simulink model "ObjectTrackerHDL_ew"  (R2024b)
settings: Solver=VariableStepAuto  StartTime=0.0  StopTime=0.2  RelTol=1e-3  EnableMultiTasking=on
PreLoadFcn:
  | % Blank input
  | img = zeros(480,640);
  | 
  | % Initialize ROI and its center
  | ROI = [175 270 127 127];
  | center = [ROI(2)+(ROI(4)+1)/2 ROI(1)+(ROI(3)+1)/2];
  | 
  | % Template Size
  | templateSize = 128;
  | tSize = templateSize;
  | 
  | % Learning rate
  | eta = 0.075;
  | 
  | % Number of training images
  | trainCount = 2;
  | 
  | % Gaussian Variance
  | sig = 2;
  | 
  | % Generate a Gaussian centered on the first frame
  | iSize = size(img);
  | [x,y] = ndgrid(1:iSize(1), 1:iSize(2));
  | gauss = exp(-((x-center(1)).^2 + (y-center(2)).^2)./(2*sig));
  | gauss = mat2gray(gauss);
  | 
  | % Generate the first template
  | img = imcrop(img, ROI);
  | gauss = imcrop(gauss, ROI);
  | 
  | % Generate the preprocess windowing function
  | [w1,w2] = meshgrid(window(@hann,tSize),window(@hann,tSize));
  | win = w1.*w2;
  | 
  | % Blank initial coefficients
  | G = zeros(tSize,tSize);
  | Ai = zeros(tSize,tSize);
  | Bi = zeros(tSize,tSize);
  | Hi = zeros(tSize,tSize);
  | 
  | numRows = tSize;
  | numCols = tSize;
InitFcn:
  | % Read the first frame
  | vidFReader = VideoReader(get_param('ObjectTrackerHDL/Input','inputFilename'));
  | img = read(vidFReader,1);
  | if (size(img,3) == 3)
  |     img = rgb2gray(img);
  | end
  | img = double(img);
  | 
  | % Initialize Object Center
  | objectCenter = str2num(get_param('ObjectTrackerHDL/ObjectTrackerHDL','objectCenter'));
  | 
  | % Template Size
  | templateSize = str2num(get_param('ObjectTrackerHDL/ObjectTrackerHDL','templateSize'));
  | originROI = objectCenter-templateSize/2;
  | tSize = templateSize;
  | 
  | % Initialize ROI and its center
  | ROI = [originROI tSize-1 tSize-1];
  | center = [ROI(2)+(ROI(4)+1)/2 ROI(1)+(ROI(3)+1)/2];
  | 
  | % Learning rate
  | eta = 0.075;
  | 
  | % Number of training images
  | trainCount = 128;
  | 
  | % Gaussian Variance
  | sig = 2;
  | 
  | % Generate a Gaussian centered on the first frame
  | iSize = size(img);
  | [x,y] = ndgrid(1:iSize(1), 1:iSize(2));
  | gauss = exp(-((x-center(1)).^2 + (y-center(2)).^2)./(2*sig));
  | gauss = mat2gray(gauss);
  | 
  | % Generate the first template
  | img = imcrop(img, ROI);
  | gauss = imcrop(gauss, ROI);
  | 
  | % Generate the preprocess windowing function
  | [w1,w2] = meshgrid(window(@hann,tSize),window(@hann,tSize));
  | win = w1.*w2;
  | 
  | % Preprocessing the first template
  | hgamma = vision.GammaCorrector(2.0,'Correction','De-gamma');
  | img = hgamma(uint8(img));
  | img = double(img);
  | mean1 = mean(img(:));
  | std1 = std(img(:));
  | img = (img-mean1)/std1;
  | fii = img.*win;
  | 
  | % Convert to frequency domain and calculate initial coefficients
  | G = fft2(gauss);
  | Ai = (G.*conj(fft2(fii)));
  | Bi = real((fft2(fii).*conj(fft2(fii))));
  | 
  | rng('default');
  | % Initial training procedure
  | for i = 1:trainCount
  | ... (+19 lines)
model workspace (MAT data in the model file):
  mwTaskManagerKernelLatency = 0
undefined symbols (not defined in the file): a, b, c, Rec, SDTV
libraries: hdlsllib x61, simulink x17, visionhdlutilities x8, visionstatistics x6, dsphdlxfrm2 x6, visionconversions x4, visiontransforms x3, visionhdlio x2, visionhdlconversions x2, visionhdlstatistics x2, visionanalysis x2, visionsinks x1
(part 2 of 3)

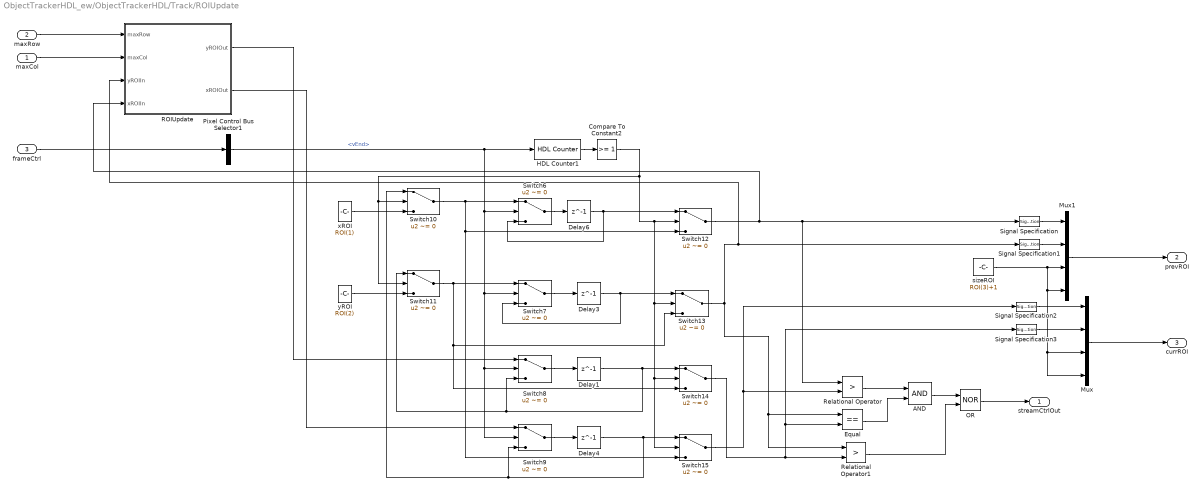
== system ObjectTrackerHDL_ew/ObjectTrackerHDL/Track/ROIUpdate ==
  maxCol : Inport
  maxRow : Inport  Port=2
  frameCtrl : Inport  Port=3
  AND : Logic  AllPortsSameDT=off  OutDataTypeStr=boolean
  Compare To Constant2 : simulink/Logic and Bit Operations/Compare To Constant  relop=>=  const=1  OutDataTypeStr=boolean
  Delay{1,3..4,6} (4 alike) : Delay  DelayLength=1
  Equal : RelationalOperator  Operator===  OutDataTypeStr=boolean  RndMeth=Simplest  InputSameDT=off
  HDL Counter1 : hdlsllib/Sources/HDL Counter  CountType=Count limited  CountInit=0  CountStep=1  CountMax=4095  CountFromType=Initial value  CountFrom=0  CountResetPort=off  CountLoadPort=off  CountEnbPort=on  CountDirPort=off  CountHitOutputPort=off  CountDataType=Unsigned  CountWordLen=12  CountFracLen=0  CountSampTime=1
  Mux : Mux
  Mux1 : Mux
  OR : Logic  Operator=NOR  AllPortsSameDT=off  OutDataTypeStr=boolean
  Pixel Control Bus Selector1 : BusSelector  OutputSignals=vEnd
  ROIUpdate : Subsystem
  Relational Operator : RelationalOperator  Operator=>  OutDataTypeStr=boolean  RndMeth=Simplest  InputSameDT=off
  Relational Operator1 : RelationalOperator  Operator=>  OutDataTypeStr=boolean  RndMeth=Simplest  InputSameDT=off
  Signal Specification{,1..3} (4 alike) : SignalSpecification  Dimensions=1
  Switch{6..15} (10 alike) : Switch  Criteria=u2 ~= 0  SaturateOnIntegerOverflow=off  InputSameDT=off
  sizeROI : Constant  Value=ROI(3)+1  OutDataTypeStr=uint16  SampleTime=-1
  xROI : Constant  Value=ROI(1)  OutDataTypeStr=uint16  SampleTime=-1
  yROI : Constant  Value=ROI(2)  OutDataTypeStr=uint16  SampleTime=-1
  streamCtrlOut : Outport
  prevROI : Outport  Port=2
  currROI : Outport  Port=3
  wires:
  Signal Specification/1 -> Mux1/1
  Switch15/1 -> Signal Specification2/1, Relational Operator/2
  Pixel Control Bus Selector1/1 -> Switch9/2, Switch8/2, Switch7/2, Switch6/2, HDL Counter1/1  "<vEnd>"
  Switch13/1 -> ROIUpdate/3(yROIIn), Signal Specification1/1, Equal/1, Relational Operator1/1
  Relational Operator/1 -> AND/1
  Signal Specification1/1 -> Mux1/2
  Switch12/1 -> ROIUpdate/4(xROIIn), Signal Specification/1, Relational Operator/1
  xROI/1 -> Switch10/3
  AND/1 -> OR/1
  Signal Specification3/1 -> Mux/2
  yROI/1 -> Switch11/3
  Switch14/1 -> Signal Specification3/1, Equal/2, Relational Operator1/2
  HDL Counter1/1 -> Compare To Constant2/1
  Equal/1 -> AND/2
  Signal Specification2/1 -> Mux/1
  Switch10/1 -> Switch15/3, Switch12/3, Switch6/1
  Relational Operator1/1 -> OR/2
  OR/1 -> streamCtrlOut/1
  maxRow/1 -> ROIUpdate/1(maxRow)
  maxCol/1 -> ROIUpdate/2(maxCol)
  Mux1/1 -> prevROI/1
  Mux/1 -> currROI/1
  Switch11/1 -> Switch14/3, Switch13/3, Switch7/1
  sizeROI/1 -> Mux/3, Mux/4, Mux1/4, Mux1/3
  Switch6/1 -> Delay6/1
  Switch7/1 -> Delay3/1
  Switch8/1 -> Delay1/1
  Switch9/1 -> Delay4/1
  Compare To Constant2/1 -> Switch12/2, Switch13/2, Switch15/2, Switch14/2, Switch11/2, Switch10/2
  frameCtrl/1 -> Pixel Control Bus Selector1/1
  Delay6/1 -> Switch6/3, Switch12/1
  Delay3/1 -> Switch7/3, Switch13/1
  Delay1/1 -> Switch8/3, Switch11/1, Switch14/1
  Delay4/1 -> Switch10/1, Switch9/3, Switch15/1
  ROIUpdate/2(xROIOut) -> Switch9/1
  ROIUpdate/1(yROIOut) -> Switch8/1

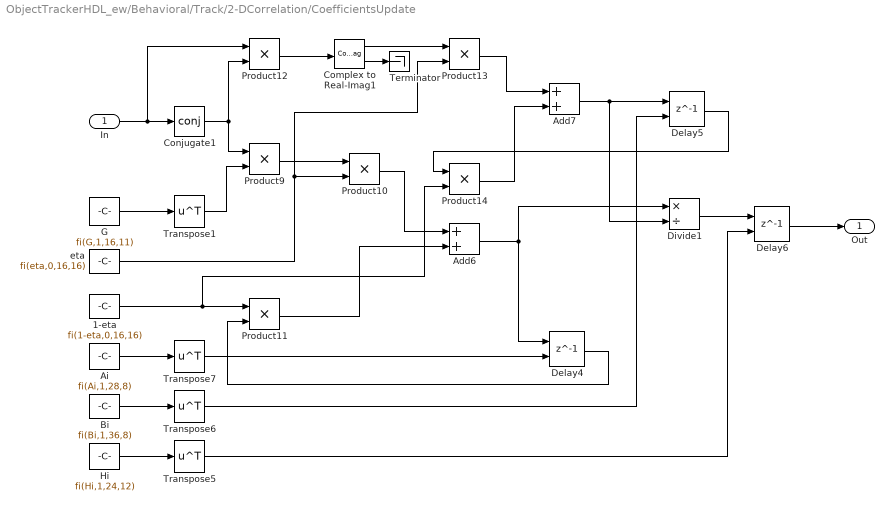
== system ObjectTrackerHDL_ew/Behavioral/Track/2-DCorrelation/CoefficientsUpdate ==
  In : Inport
  1-eta : Constant  Value=fi(1-eta,0,16,16)  OutDataTypeStr=fixdt(0,16,16)  SampleTime=-1
  Add6 : Sum  OutDataTypeStr=fixdt(1,28,8)
  Add7 : Sum  OutDataTypeStr=fixdt(1,36,8)
  Ai : Constant  Value=fi(Ai,1,28,8)  OutDataTypeStr=fixdt(1,28,8)  SampleTime=-1
  Bi : Constant  Value=fi(Bi,1,36,8)  OutDataTypeStr=fixdt(1,36,8)  SampleTime=-1
  Complex to Real-Imag1 : ComplexToRealImag
  Conjugate1 : Math  Operator=conj  SignedPower=on  RndMeth=Zero
  Delay4 : Delay  DelayLength=1  InitialConditionSource=Input port  InitialCondition=Ai
      settings: InputPortMap=u0,p4
  Delay5 : Delay  DelayLength=1  InitialConditionSource=Input port  InitialCondition=Bi
      settings: InputPortMap=u0,p4
  Delay6 : Delay  DelayLength=1  InitialConditionSource=Input port  InitialCondition=Hi
      settings: InputPortMap=u0,p4
  Divide1 : Product  Inputs=*/  OutDataTypeStr=fixdt(1,24,12)  RndMeth=Simplest  SaturateOnIntegerOverflow=on
  G : Constant  Value=fi(G,1,16,11)  VectorParams1D=off  SampleTime=-1
  Hi : Constant  Value=fi(Hi,1,24,12)  OutDataTypeStr=fixdt(1,24,12)  SampleTime=-1
  Product10 : Product  OutDataTypeStr=fixdt(1,24,12)
  Product11 : Product  OutDataTypeStr=fixdt(1,28,8)
  Product12 : Product  OutDataTypeStr=fixdt(1,32,8)
  Product13 : Product  OutDataTypeStr=fixdt(1,32,12)
  Product14 : Product  OutDataTypeStr=fixdt(1,36,8)
  Product9 : Product  OutDataTypeStr=fixdt(1,24,8)
  Terminator : Terminator
  Transpose{1,5..7} (4 alike) : Math  Operator=transpose
  eta : Constant  Value=fi(eta,0,16,16)  SampleTime=-1
  Out : Outport
  wires:
  Product14/1 -> Add7/2
  Ai/1 -> Transpose7/1
  Add6/1 -> Delay4/1, Divide1/1
  Divide1/1 -> Delay6/1
  eta/1 -> Product13/2, Product10/2
  In/1 -> Product12/1, Conjugate1/1
  Product9/1 -> Product10/1
  Conjugate1/1 -> Product12/2, Product9/1
  Product11/1 -> Add6/2
  1-eta/1 -> Product11/1, Product14/2
  Transpose6/1 -> Delay5/2
  Add7/1 -> Delay5/1, Divide1/2
  Hi/1 -> Transpose5/1
  Product10/1 -> Add6/1
  Delay5/1 -> Product14/1
  Product13/1 -> Add7/1
  G/1 -> Transpose1/1
  Complex to Real-Imag1/2 -> Terminator/1
  Complex to Real-Imag1/1 -> Product13/1
  Delay6/1 -> Out/1
  Bi/1 -> Transpose6/1
  Product12/1 -> Complex to Real-Imag1/1
  Transpose5/1 -> Delay6/2
  Transpose7/1 -> Delay4/2
  Delay4/1 -> Product11/2
  Transpose1/1 -> Product9/2

== system ObjectTrackerHDL_ew/Behavioral/Track/ROIUpdate/CurrValidROI ==
  ROIIn : Inport
  Constant : Constant  Value=iSize(1)-tSize  OutDataTypeStr=uint16  SampleTime=-1
  Constant1 : Constant  Value=iSize(2)-tSize  OutDataTypeStr=uint16  SampleTime=-1
  Demux : Demux
  Mux1 : Mux
  Relational Operator : RelationalOperator  Operator=<  OutDataTypeStr=boolean  RndMeth=Simplest  InputSameDT=off
  Relational Operator1 : RelationalOperator  Operator=<  OutDataTypeStr=boolean  RndMeth=Simplest  InputSameDT=off
  Switch : Switch  Criteria=u2 ~= 0  SaturateOnIntegerOverflow=off  InputSameDT=off
  Switch1 : Switch  Criteria=u2 ~= 0  SaturateOnIntegerOverflow=off  InputSameDT=off
  ROIOut : Outport
  wires:
  Mux1/1 -> ROIOut/1
  ROIIn/1 -> Demux/1
  Demux/1 -> Switch/1, Relational Operator/1
  Constant1/1 -> Switch/3, Relational Operator/2
  Demux/2 -> Relational Operator1/1, Switch1/1
  Constant/1 -> Switch1/3, Relational Operator1/2
  Demux/3 -> Mux1/3
  Demux/4 -> Mux1/4
  Relational Operator/1 -> Switch/2
  Switch/1 -> Mux1/1
  Relational Operator1/1 -> Switch1/2
  Switch1/1 -> Mux1/2

== system ObjectTrackerHDL_ew/Behavioral/Track/ROIUpdate/PrevValidROI ==
  ROIIn : Inport
  Constant : Constant  Value=iSize(1)-tSize  OutDataTypeStr=uint16  SampleTime=-1
  Constant1 : Constant  Value=iSize(2)-tSize  OutDataTypeStr=uint16  SampleTime=-1
  Demux : Demux
  Mux1 : Mux
  Relational Operator : RelationalOperator  Operator=<  OutDataTypeStr=boolean  RndMeth=Simplest  InputSameDT=off
  Relational Operator1 : RelationalOperator  Operator=<  OutDataTypeStr=boolean  RndMeth=Simplest  InputSameDT=off
  Switch : Switch  Criteria=u2 ~= 0  SaturateOnIntegerOverflow=off  InputSameDT=off
  Switch1 : Switch  Criteria=u2 ~= 0  SaturateOnIntegerOverflow=off  InputSameDT=off
  ROIOut : Outport
  wires:
  Mux1/1 -> ROIOut/1
  ROIIn/1 -> Demux/1
  Demux/1 -> Switch/1, Relational Operator/1
  Constant1/1 -> Switch/3, Relational Operator/2
  Demux/2 -> Relational Operator1/1, Switch1/1
  Constant/1 -> Switch1/3, Relational Operator1/2
  Demux/3 -> Mux1/3
  Demux/4 -> Mux1/4
  Relational Operator/1 -> Switch/2
  Switch/1 -> Mux1/1
  Relational Operator1/1 -> Switch1/2
  Switch1/1 -> Mux1/2

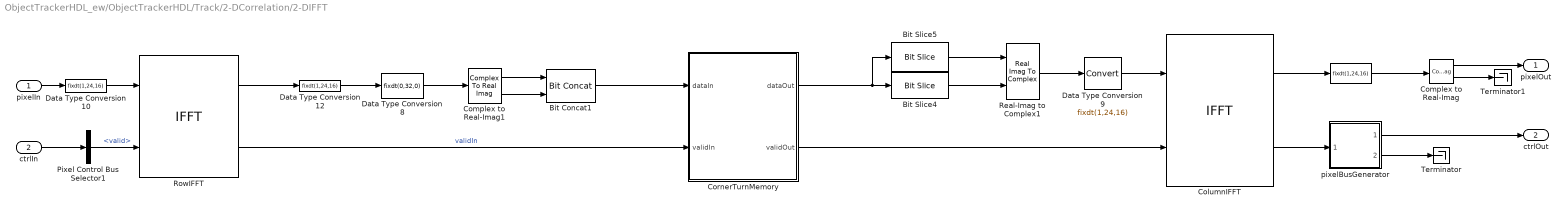
== system ObjectTrackerHDL_ew/ObjectTrackerHDL/Track/2-DCorrelation/2-DIFFT ==
  pixelIn : Inport
  ctrlIn : Inport  Port=2
  " " : DataTypeConversion  OutDataTypeStr=fixdt(1,24,16)  SaturateOnIntegerOverflow=off  RndMeth=Floor
  Bit Concat1 : hdlsllib/Logic and Bit Operations/Bit Concat  numInputs=2
  Bit Slice4 : hdlsllib/Logic and Bit Operations/Bit Slice  lidx=31  ridx=0
  Bit Slice5 : hdlsllib/Logic and Bit Operations/Bit Slice  lidx=63  ridx=32
  ColumnIFFT : dsphdlxfrm2/IFFT  Architecture=Streaming Radix 2^2  FFTLengthSource=Property  FFTLength=tSize  FFTLengthMax=1024  ComplexMultiplication=Use 4 multipliers and 2 adders  BitReversedOutput=off  BitReversedInput=off  Normalize=on  SimulateUsing=Code generation  RoundingMethod=Floor  ResetInputPort=off  StartOutputPort=off  EndOutputPort=off
  Complex to Real-Imag : ComplexToRealImag
  Complex to Real-Imag1 : ComplexToRealImag
  CornerTurnMemory : Subsystem
  Data Type Conversion10 : DataTypeConversion  OutDataTypeStr=fixdt(1,24,16)  SaturateOnIntegerOverflow=off  RndMeth=Floor
  Data Type Conversion12 : DataTypeConversion  OutDataTypeStr=fixdt(1,24,16)  SaturateOnIntegerOverflow=off  RndMeth=Floor
  Data Type Conversion8 : DataTypeConversion  OutDataTypeStr=fixdt(0,32,0)  ConvertRealWorld=Stored Integer (SI)  SaturateOnIntegerOverflow=off  RndMeth=Floor
  Data Type Conversion9 : DataTypeConversion  OutDataTypeStr=fixdt(1,24,16)  ConvertRealWorld=Stored Integer (SI)  SaturateOnIntegerOverflow=off  RndMeth=Floor
  Pixel Control Bus Selector1 : BusSelector  OutputSignals=valid
  Real-Imag to Complex1 : RealImagToComplex
  RowIFFT : dsphdlxfrm2/IFFT  Architecture=Streaming Radix 2^2  FFTLengthSource=Property  FFTLength=tSize  FFTLengthMax=1024  ComplexMultiplication=Use 4 multipliers and 2 adders  BitReversedOutput=off  BitReversedInput=off  Normalize=on  SimulateUsing=Code generation  RoundingMethod=Floor  ResetInputPort=off  StartOutputPort=off  EndOutputPort=off
  Terminator : Terminator
  Terminator1 : Terminator
  pixelBusGenerator : Subsystem  mask{hEnd=tSize - 1, vEnd=tSize * tSize - 1}
      mask prompts: hEnd "hEnd Count"; vEnd "vEnd Count"
      mask DialogControl DescGroupVar Prompt: Counter Values
  pixelOut : Outport
  ctrlOut : Outport  Port=2
  wires:
  Bit Slice4/1 -> Real-Imag to Complex1/2
  Complex to Real-Imag1/1 -> Bit Concat1/1
  pixelIn/1 -> Data Type Conversion10/1
  Data Type Conversion12/1 -> Data Type Conversion8/1
  Data Type Conversion8/1 -> Complex to Real-Imag1/1
  Data Type Conversion10/1 -> RowIFFT/1
  ColumnIFFT/1 -> " "/1
  ctrlIn/1 -> Pixel Control Bus Selector1/1
  pixelBusGenerator/2(frameDone) -> Terminator/1
  RowIFFT/1 -> Data Type Conversion12/1
  Complex to Real-Imag1/2 -> Bit Concat1/2
  ColumnIFFT/2 -> pixelBusGenerator/1(validIn)
  Data Type Conversion9/1 -> ColumnIFFT/1
  Bit Slice5/1 -> Real-Imag to Complex1/1
  Real-Imag to Complex1/1 -> Data Type Conversion9/1
  pixelBusGenerator/1(busOut) -> ctrlOut/1
  " "/1 -> Complex to Real-Imag/1
  Complex to Real-Imag/1 -> pixelOut/1
  Complex to Real-Imag/2 -> Terminator1/1
  Pixel Control Bus Selector1/1 -> RowIFFT/2  "<valid>"
  CornerTurnMemory/1(dataOut) -> Bit Slice5/1, Bit Slice4/1
  Bit Concat1/1 -> CornerTurnMemory/1(dataIn)
  RowIFFT/2 -> CornerTurnMemory/2(validIn)  "validIn"
  CornerTurnMemory/2(validOut) -> ColumnIFFT/2

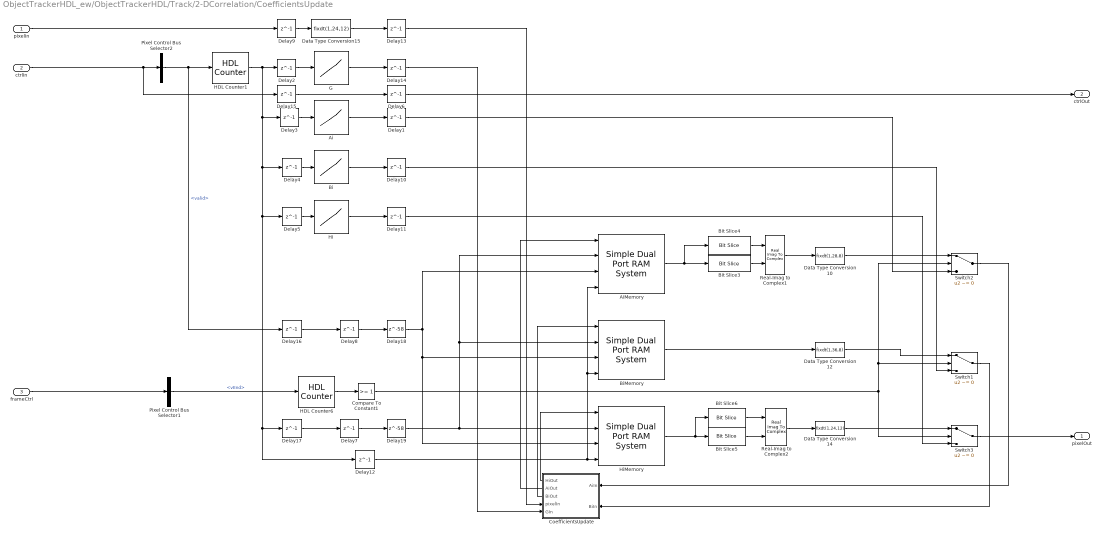
== system ObjectTrackerHDL_ew/ObjectTrackerHDL/Track/2-DCorrelation/CoefficientsUpdate ==
  pixelIn : Inport
  ctrlIn : Inport  Port=2
  frameCtrl : Inport  Port=3
  Ai : Lookup_n-D  NumberOfTableDimensions=1  LookupTableObject=''  BreakpointsForDimension1=[0:tSize * tSize - 1]  BreakpointsForDimension1FirstPoint=10  BreakpointsForDimension2FirstPoint=10  BreakpointsForDimension1Spacing=12  BreakpointsForDimension2Spacing=12  IndexSearchMethod=Evenly spaced points  Table=fi(Ai(:),1,28,8)  InterpMethod=Flat  DiagnosticForOutOfRangeInput=Error  InternalRulePriority=Speed  OutDataTypeStr=fixdt(1,28,8)  RndMeth=Simplest
  AiMemory : hdlsllib/HDL RAMs/Simple Dual Port RAM System  RAMType=Simple dual port  AsyncRead=off  WriteOutputValue=New data  RAMInitialValue=0  allowBusInputs=off  WritesHaveOutput=on  NumReads=0  NumWrites=1  SimulateUsing=Code generation  ModelRAMDelay=on
  Bi : Lookup_n-D  NumberOfTableDimensions=1  LookupTableObject=''  BreakpointsForDimension1=[0:tSize * tSize - 1]  BreakpointsForDimension1FirstPoint=10  BreakpointsForDimension2FirstPoint=10  BreakpointsForDimension1Spacing=12  BreakpointsForDimension2Spacing=12  IndexSearchMethod=Evenly spaced points  Table=fi(Bi(:),1,36,8)  InterpMethod=Flat  DiagnosticForOutOfRangeInput=Error  InternalRulePriority=Speed  OutDataTypeStr=fixdt(1,36,8)  RndMeth=Simplest
  BiMemory : hdlsllib/HDL RAMs/Simple Dual Port RAM System  RAMType=Simple dual port  AsyncRead=off  WriteOutputValue=New data  RAMInitialValue=0  allowBusInputs=off  WritesHaveOutput=on  NumReads=0  NumWrites=1  SimulateUsing=Code generation  ModelRAMDelay=on
  Bit Slice3 : hdlsllib/Logic and Bit Operations/Bit Slice  lidx=31  ridx=0
  Bit Slice4 : hdlsllib/Logic and Bit Operations/Bit Slice  lidx=63  ridx=32
  Bit Slice5 : hdlsllib/Logic and Bit Operations/Bit Slice  lidx=31  ridx=0
  Bit Slice6 : hdlsllib/Logic and Bit Operations/Bit Slice  lidx=63  ridx=32
  CoefficientsUpdate : Subsystem
      settings: PortSchema="{\"entries\":[{\"content\":{\"sides\":[{\"content\":{\"connectorIds\":[\"Out1\",\"Out2\",\"Out3\",\"In1\",\"In2\"]},\"type\":\"ConnectorPlacement.EquallySpacedRectSide\",\"uuid\":\"191c5b09-aed9-4d47-87b5-72a6c40c9cca\"},{\"content\":{\"connectorIds\":[\"In3\",\"In4\"],\"side\":\"RIGHT\"},\"type\":\"ConnectorPlacement.EquallySpacedRectSide\",\"uuid\":\"decd93cb-43a4-41cc-87f2-68ffa8f89900\"},{\"content\":{\"side\":\"TOP\"},\"type\":\"ConnectorPlacement.EquallySpacedRectSide\",\"uuid\":\"0d8c8ea6-6c17-441a-9a0f-239b887dcd47\"}]},\"type\":\"ConnectorPlacement.EquallySpacedConnector\",\"uuid\":\"0ec76fdc-f9ed-4753-8274-de70c3f7ff2d\"}],\"packageUris\":[\"http://schema.mathworks.com/mf0/Connector/R2020b\"],\"version\":\"1.0\"}"
  Compare To Constant1 : simulink/Logic and Bit Operations/Compare To Constant  relop=>=  const=1  OutDataTypeStr=boolean
  Data Type Conversion10 : DataTypeConversion  OutDataTypeStr=fixdt(1,28,8)  ConvertRealWorld=Stored Integer (SI)  SaturateOnIntegerOverflow=off  RndMeth=Floor
  Data Type Conversion12 : DataTypeConversion  OutDataTypeStr=fixdt(1,36,8)  ConvertRealWorld=Stored Integer (SI)  SaturateOnIntegerOverflow=off  RndMeth=Floor
  Data Type Conversion14 : DataTypeConversion  OutDataTypeStr=fixdt(1,24,12)  ConvertRealWorld=Stored Integer (SI)  SaturateOnIntegerOverflow=off  RndMeth=Floor
  Data Type Conversion15 : DataTypeConversion  OutDataTypeStr=fixdt(1,24,12)  SaturateOnIntegerOverflow=off  RndMeth=Floor
  Delay{1..17} (17 alike) : Delay  DelayLength=1
  Delay18 : Delay  DelayLength=58
  Delay19 : Delay  DelayLength=58
  G : Lookup_n-D  NumberOfTableDimensions=1  LookupTableObject=''  BreakpointsForDimension1=[0:tSize * tSize - 1]  BreakpointsForDimension1FirstPoint=10  BreakpointsForDimension2FirstPoint=10  BreakpointsForDimension1Spacing=12  BreakpointsForDimension2Spacing=12  IndexSearchMethod=Evenly spaced points  Table=fi(G(:),1,16,11)  InterpMethod=Flat  DiagnosticForOutOfRangeInput=Error  InternalRulePriority=Speed  OutDataTypeStr=fixdt(1,16,11)  RndMeth=Simplest
  HDL Counter1 : hdlsllib/Sources/HDL Counter  CountType=Count limited  CountInit=0  CountStep=1  CountMax=tSize * tSize - 1  CountFromType=Initial value  CountFrom=0  CountResetPort=off  CountLoadPort=off  CountEnbPort=on  CountDirPort=off  CountHitOutputPort=off  CountDataType=Unsigned  CountWordLen=ceil(log2(tSize * tSize - 1))  CountFracLen=0  CountSampTime=1
  HDL Counter6 : hdlsllib/Sources/HDL Counter  CountType=Count limited  CountInit=0  CountStep=1  CountMax=4095  CountFromType=Initial value  CountFrom=0  CountResetPort=off  CountLoadPort=off  CountEnbPort=on  CountDirPort=off  CountHitOutputPort=off  CountDataType=Unsigned  CountWordLen=12  CountFracLen=0  CountSampTime=1
  Hi : Lookup_n-D  NumberOfTableDimensions=1  LookupTableObject=''  BreakpointsForDimension1=[0:tSize * tSize - 1]  BreakpointsForDimension1FirstPoint=10  BreakpointsForDimension2FirstPoint=10  BreakpointsForDimension1Spacing=12  BreakpointsForDimension2Spacing=12  IndexSearchMethod=Evenly spaced points  Table=fi(Hi(:),1,24,12)  InterpMethod=Flat  DiagnosticForOutOfRangeInput=Error  InternalRulePriority=Speed  OutDataTypeStr=fixdt(1,24,12)  RndMeth=Simplest
  HiMemory : hdlsllib/HDL RAMs/Simple Dual Port RAM System  RAMType=Simple dual port  AsyncRead=off  WriteOutputValue=New data  RAMInitialValue=0  allowBusInputs=off  WritesHaveOutput=on  NumReads=0  NumWrites=1  SimulateUsing=Code generation  ModelRAMDelay=on
  Pixel Control Bus Selector1 : BusSelector  OutputSignals=vEnd
  Pixel Control Bus Selector2 : BusSelector  OutputSignals=valid
  Real-Imag to Complex1 : RealImagToComplex
  Real-Imag to Complex2 : RealImagToComplex
  Switch1 : Switch  Criteria=u2 ~= 0  SaturateOnIntegerOverflow=off  InputSameDT=off
  Switch2 : Switch  Criteria=u2 ~= 0  SaturateOnIntegerOverflow=off  InputSameDT=off
  Switch3 : Switch  Criteria=u2 ~= 0  SaturateOnIntegerOverflow=off  InputSameDT=off
  pixelOut : Outport
  ctrlOut : Outport  Port=2
  wires:
  Delay7/1 -> Delay19/1
  Data Type Conversion12/1 -> Switch1/1
  Bit Slice5/1 -> Real-Imag to Complex2/2
  AiMemory/1 -> Bit Slice4/1, Bit Slice3/1
  Pixel Control Bus Selector2/1 -> HDL Counter1/1, Delay16/1  "<valid>"
  Real-Imag to Complex1/1 -> Data Type Conversion10/1
  Bit Slice4/1 -> Real-Imag to Complex1/1
  Bit Slice3/1 -> Real-Imag to Complex1/2
  BiMemory/1 -> Data Type Conversion12/1
  Data Type Conversion10/1 -> Switch2/1
  HDL Counter6/1 -> Compare To Constant1/1
  Bit Slice6/1 -> Real-Imag to Complex2/1
  Real-Imag to Complex2/1 -> Data Type Conversion14/1
  Data Type Conversion15/1 -> Delay13/1
  G/1 -> Delay14/1
  Switch2/1 -> CoefficientsUpdate/3(AiIn)
  Switch1/1 -> CoefficientsUpdate/4(BiIn)
  Pixel Control Bus Selector1/1 -> HDL Counter6/1  "<vEnd>"
  HiMemory/1 -> Bit Slice5/1, Bit Slice6/1
  Compare To Constant1/1 -> Switch3/2, Switch2/2, Switch1/2
  Data Type Conversion14/1 -> Switch3/1
  Delay8/1 -> Delay18/1
  Delay2/1 -> G/1
  Delay3/1 -> Ai/1
  Delay4/1 -> Bi/1
  Delay5/1 -> Hi/1
  Delay6/1 -> ctrlOut/1
  Delay9/1 -> Data Type Conversion15/1
  ctrlIn/1 -> Delay15/1, Pixel Control Bus Selector2/1
  pixelIn/1 -> Delay9/1
  frameCtrl/1 -> Pixel Control Bus Selector1/1
  CoefficientsUpdate/1(HiOut) -> HiMemory/1
  CoefficientsUpdate/3(BiOut) -> BiMemory/1
  CoefficientsUpdate/2(AiOut) -> AiMemory/1
  HDL Counter1/1 -> Delay12/1, Delay17/1, Delay5/1, Delay4/1, Delay3/1, Delay2/1
  Switch3/1 -> pixelOut/1
  Hi/1 -> Delay11/1
  Bi/1 -> Delay10/1
  Ai/1 -> Delay1/1
  Delay1/1 -> Switch2/3
  Delay10/1 -> Switch1/3
  Delay11/1 -> Switch3/3
  Delay12/1 -> HiMemory/4, AiMemory/4, BiMemory/4
  Delay13/1 -> CoefficientsUpdate/1(pixelIn)
  Delay14/1 -> CoefficientsUpdate/2(GIn)
  Delay15/1 -> Delay6/1
  Delay16/1 -> Delay8/1
  Delay17/1 -> Delay7/1
  Delay18/1 -> BiMemory/3, HiMemory/3, AiMemory/3
  Delay19/1 -> AiMemory/2, BiMemory/2, HiMemory/2

== system ObjectTrackerHDL_ew/ObjectTrackerHDL/Track/2-DCorrelation/Curr2-DFFT ==
  pixelIn : Inport
  ctrlIn : Inport  Port=2
  " " : DataTypeConversion  OutDataTypeStr=fixdt(1,24,12)  SaturateOnIntegerOverflow=off  RndMeth=Floor
  Bit Concat : hdlsllib/Logic and Bit Operations/Bit Concat  numInputs=2
  Bit Slice1 : hdlsllib/Logic and Bit Operations/Bit Slice  lidx=31  ridx=0
  Bit Slice2 : hdlsllib/Logic and Bit Operations/Bit Slice  lidx=63  ridx=32
  ColumnFFT : dsphdlxfrm2/FFT  Architecture=Streaming Radix 2^2  FFTLengthSource=Property  FFTLength=tSize  FFTLengthMax=1024  ComplexMultiplication=Use 4 multipliers and 2 adders  BitReversedOutput=off  BitReversedInput=off  Normalize=off  SimulateUsing=Code generation  RoundingMethod=Floor  ResetInputPort=off  StartOutputPort=off  EndOutputPort=off
  Complex to Real-Imag1 : ComplexToRealImag
  CornerTurnMemory : Subsystem
  Data Type Conversion2 : DataTypeConversion  OutDataTypeStr=fixdt(0,32,0)  ConvertRealWorld=Stored Integer (SI)  SaturateOnIntegerOverflow=off  RndMeth=Floor
  Data Type Conversion3 : DataTypeConversion  OutDataTypeStr=fixdt(1,28,16)  ConvertRealWorld=Stored Integer (SI)  SaturateOnIntegerOverflow=off  RndMeth=Floor
  Data Type Conversion6 : DataTypeConversion  OutDataTypeStr=fixdt(1,28,16)  SaturateOnIntegerOverflow=off  RndMeth=Floor
  Pixel Control Bus Selector1 : BusSelector  OutputSignals=valid
  Real-Imag to Complex : RealImagToComplex
  RowFFT : dsphdlxfrm2/FFT  Architecture=Streaming Radix 2^2  FFTLengthSource=Property  FFTLength=tSize  FFTLengthMax=1024  ComplexMultiplication=Use 4 multipliers and 2 adders  BitReversedOutput=off  BitReversedInput=off  Normalize=off  SimulateUsing=Code generation  RoundingMethod=Floor  ResetInputPort=off  StartOutputPort=off  EndOutputPort=off
  Terminator : Terminator
  pixelBusGenerator : Subsystem  mask{hEnd=tSize - 1, vEnd=tSize * tSize - 1}
      mask prompts: hEnd "hEnd Count"; vEnd "vEnd Count"
      mask DialogControl DescGroupVar Prompt: Counter Values
  pixelOut : Outport
  ctrlOut : Outport  Port=2
  wires:
  Data Type Conversion3/1 -> ColumnFFT/1
  pixelIn/1 -> RowFFT/1
  Data Type Conversion6/1 -> Data Type Conversion2/1
  ColumnFFT/2 -> pixelBusGenerator/1(validIn)
  Pixel Control Bus Selector1/1 -> RowFFT/2  "<valid>"
  RowFFT/1 -> Data Type Conversion6/1
  Bit Slice2/1 -> Real-Imag to Complex/1
  Real-Imag to Complex/1 -> Data Type Conversion3/1
  pixelBusGenerator/1(busOut) -> ctrlOut/1
  Complex to Real-Imag1/2 -> Bit Concat/2
  Data Type Conversion2/1 -> Complex to Real-Imag1/1
  Complex to Real-Imag1/1 -> Bit Concat/1
  Bit Slice1/1 -> Real-Imag to Complex/2
  " "/1 -> pixelOut/1
  ColumnFFT/1 -> " "/1
  ctrlIn/1 -> Pixel Control Bus Selector1/1
  pixelBusGenerator/2(frameDone) -> Terminator/1
  CornerTurnMemory/1(dataOut) -> Bit Slice1/1, Bit Slice2/1
  Bit Concat/1 -> CornerTurnMemory/1(dataIn)
  RowFFT/2 -> CornerTurnMemory/2(validIn)
  CornerTurnMemory/2(validOut) -> ColumnFFT/2

== system ObjectTrackerHDL_ew/ObjectTrackerHDL/Track/2-DCorrelation/Prev2-DFFT ==
  pixelIn : Inport
  ctrlIn : Inport  Port=2
  " " : DataTypeConversion  OutDataTypeStr=fixdt(1,24,12)  SaturateOnIntegerOverflow=off  RndMeth=Floor
  Bit Concat : hdlsllib/Logic and Bit Operations/Bit Concat  numInputs=2
  Bit Slice1 : hdlsllib/Logic and Bit Operations/Bit Slice  lidx=31  ridx=0
  Bit Slice2 : hdlsllib/Logic and Bit Operations/Bit Slice  lidx=63  ridx=32
  ColumnFFT : dsphdlxfrm2/FFT  Architecture=Streaming Radix 2^2  FFTLengthSource=Property  FFTLength=tSize  FFTLengthMax=1024  ComplexMultiplication=Use 4 multipliers and 2 adders  BitReversedOutput=off  BitReversedInput=off  Normalize=off  SimulateUsing=Code generation  RoundingMethod=Floor  ResetInputPort=off  StartOutputPort=off  EndOutputPort=off
  Complex to Real-Imag1 : ComplexToRealImag
  CornerTurnMemory : Subsystem
  Data Type Conversion2 : DataTypeConversion  OutDataTypeStr=fixdt(0,32,0)  ConvertRealWorld=Stored Integer (SI)  SaturateOnIntegerOverflow=off  RndMeth=Floor
  Data Type Conversion3 : DataTypeConversion  OutDataTypeStr=fixdt(1,28,16)  ConvertRealWorld=Stored Integer (SI)  SaturateOnIntegerOverflow=off  RndMeth=Floor
  Data Type Conversion6 : DataTypeConversion  OutDataTypeStr=fixdt(1,28,16)  SaturateOnIntegerOverflow=off  RndMeth=Floor
  Pixel Control Bus Selector1 : BusSelector  OutputSignals=valid
  Real-Imag to Complex : RealImagToComplex
  RowFFT : dsphdlxfrm2/FFT  Architecture=Streaming Radix 2^2  FFTLengthSource=Property  FFTLength=tSize  FFTLengthMax=1024  ComplexMultiplication=Use 4 multipliers and 2 adders  BitReversedOutput=off  BitReversedInput=off  Normalize=off  SimulateUsing=Code generation  RoundingMethod=Floor  ResetInputPort=off  StartOutputPort=off  EndOutputPort=off
  Terminator : Terminator
  pixelBusGenerator : Subsystem  mask{hEnd=tSize - 1, vEnd=tSize * tSize - 1}
      mask prompts: hEnd "hEnd Count"; vEnd "vEnd Count"
      mask DialogControl DescGroupVar Prompt: Counter Values
  pixelOut : Outport
  ctrlOut : Outport  Port=2
  wires:
  Data Type Conversion3/1 -> ColumnFFT/1
  pixelIn/1 -> RowFFT/1
  Data Type Conversion6/1 -> Data Type Conversion2/1
  ColumnFFT/2 -> pixelBusGenerator/1(validIn)
  Pixel Control Bus Selector1/1 -> RowFFT/2  "<valid>"
  RowFFT/1 -> Data Type Conversion6/1
  Bit Slice2/1 -> Real-Imag to Complex/1
  Real-Imag to Complex/1 -> Data Type Conversion3/1
  pixelBusGenerator/1(busOut) -> ctrlOut/1
  Complex to Real-Imag1/2 -> Bit Concat/2
  Data Type Conversion2/1 -> Complex to Real-Imag1/1
  Complex to Real-Imag1/1 -> Bit Concat/1
  Bit Slice1/1 -> Real-Imag to Complex/2
  " "/1 -> pixelOut/1
  ColumnFFT/1 -> " "/1
  ctrlIn/1 -> Pixel Control Bus Selector1/1
  pixelBusGenerator/2(frameDone) -> Terminator/1
  CornerTurnMemory/1(dataOut) -> Bit Slice2/1, Bit Slice1/1
  Bit Concat/1 -> CornerTurnMemory/1(dataIn)
  RowFFT/2 -> CornerTurnMemory/2(validIn)
  CornerTurnMemory/2(validOut) -> ColumnFFT/2

== system ObjectTrackerHDL_ew/ObjectTrackerHDL/Track/2-DCorrelation/StreamAlignment ==
  pixelIn1 : Inport
  ctrlIn1 : Inport  Port=2
  pixelIn2 : Inport  Port=3
  ctrlIn2 : Inport  Port=4
  streamCtrl : Inport  Port=5
  Complex to Real-Imag : ComplexToRealImag
  Complex to Real-Imag1 : ComplexToRealImag
  Pixel Stream Aligner : visionhdlutilities/Pixel Stream Aligner  LineBufferSize=256  MaximumNumberOfLines=tSize  SimulateUsing=Code generation
  Pixel Stream Aligner1 : visionhdlutilities/Pixel Stream Aligner  LineBufferSize=256  MaximumNumberOfLines=tSize  SimulateUsing=Code generation
  Real-Imag to Complex : RealImagToComplex
  Real-Imag to Complex1 : RealImagToComplex
  Switch{2..5} (4 alike) : Switch  Criteria=u2 ~= 0  SaturateOnIntegerOverflow=off  InputSameDT=off
  Terminator : Terminator
  pixelOut1 : Outport
  pixelOut2 : Outport  Port=2
  ctrlOut : Outport  Port=3
  wires:
  Pixel Stream Aligner/2 -> Real-Imag to Complex1/1
  Complex to Real-Imag1/2 -> Pixel Stream Aligner1/3
  Switch4/1 -> Complex to Real-Imag1/1
  Real-Imag to Complex/1 -> pixelOut1/1
  Switch5/1 -> Pixel Stream Aligner1/4, Pixel Stream Aligner/4
  Complex to Real-Imag/1 -> Pixel Stream Aligner/1
  streamCtrl/1 -> Switch2/2, Switch3/2, Switch4/2, Switch5/2
  Pixel Stream Aligner/1 -> Real-Imag to Complex/1
  Switch3/1 -> Pixel Stream Aligner1/2, Pixel Stream Aligner/2
  pixelIn2/1 -> Switch4/1, Switch2/3
  Pixel Stream Aligner/3 -> ctrlOut/1
  ctrlIn1/1 -> Switch5/3, Switch3/1
  ctrlIn2/1 -> Switch3/3, Switch5/1
  Pixel Stream Aligner1/1 -> Real-Imag to Complex/2
  pixelIn1/1 -> Switch4/3, Switch2/1
  Switch2/1 -> Complex to Real-Imag/1
  Complex to Real-Imag/2 -> Pixel Stream Aligner1/1
  Complex to Real-Imag1/1 -> Pixel Stream Aligner/3
  Pixel Stream Aligner1/2 -> Real-Imag to Complex1/2
  Real-Imag to Complex1/1 -> pixelOut2/1
  Pixel Stream Aligner1/3 -> Terminator/1

== system ObjectTrackerHDL_ew/ObjectTrackerHDL/Track/MaxCorrelation/MaxCtrl ==
  pixelIn : Inport
  reset : Inport  Port=2
  AND : Logic  Operator=NOT  AllPortsSameDT=off  OutDataTypeStr=boolean
  AND1 : Logic  AllPortsSameDT=off  OutDataTypeStr=boolean
  AND2 : Logic  AllPortsSameDT=off  OutDataTypeStr=boolean
  Compare To Zero : simulink/Logic and Bit Operations/Compare To Zero  relop=~=  OutDataTypeStr=boolean
  Constant3 : Constant  Value=0  OutDataTypeStr=fixdt(1,24,16)  SampleTime=-1
  Delay : Delay  DelayLength=1
  Delay4 : Delay
  Delay5 : Delay
  Delay8 : Delay  DelayLength=1
  Max : MinMax  Function=max  Inputs=2
  NOT : Logic  Operator=NOT  AllPortsSameDT=off  OutDataTypeStr=boolean
  Relational Operator : RelationalOperator  Operator=~=  OutDataTypeStr=boolean  RndMeth=Simplest  InputSameDT=off
  Relational Operator1 : RelationalOperator  Operator===  OutDataTypeStr=boolean  RndMeth=Simplest  InputSameDT=off
  Switch7 : Switch  Criteria=u2 ~= 0  SaturateOnIntegerOverflow=off  InputSameDT=off
  Switch8 : Switch  Criteria=u2 ~= 0  SaturateOnIntegerOverflow=off  InputSameDT=off
  newMaxCtrl : Outport
  sameMaxCtrl : Outport  Port=2
  wires:
  Max/1 -> Relational Operator/2, Compare To Zero/1, Relational Operator1/2, Delay/1
  Switch8/1 -> Max/2
  AND2/1 -> Delay5/1
  AND1/1 -> sameMaxCtrl/1
  NOT/1 -> Delay8/1
  Delay/1 -> Switch8/1, Relational Operator/1
  Delay8/1 -> Switch8/2, Switch7/2
  Delay4/1 -> newMaxCtrl/1, AND/1
  Constant3/1 -> Switch7/3, Switch8/3
  Delay5/1 -> AND1/2
  reset/1 -> NOT/1
  Relational Operator1/1 -> AND2/1
  pixelIn/1 -> Relational Operator1/1, Switch7/1
  AND/1 -> AND1/1
  Switch7/1 -> Max/1
  Relational Operator/1 -> Delay4/1
  Compare To Zero/1 -> AND2/2

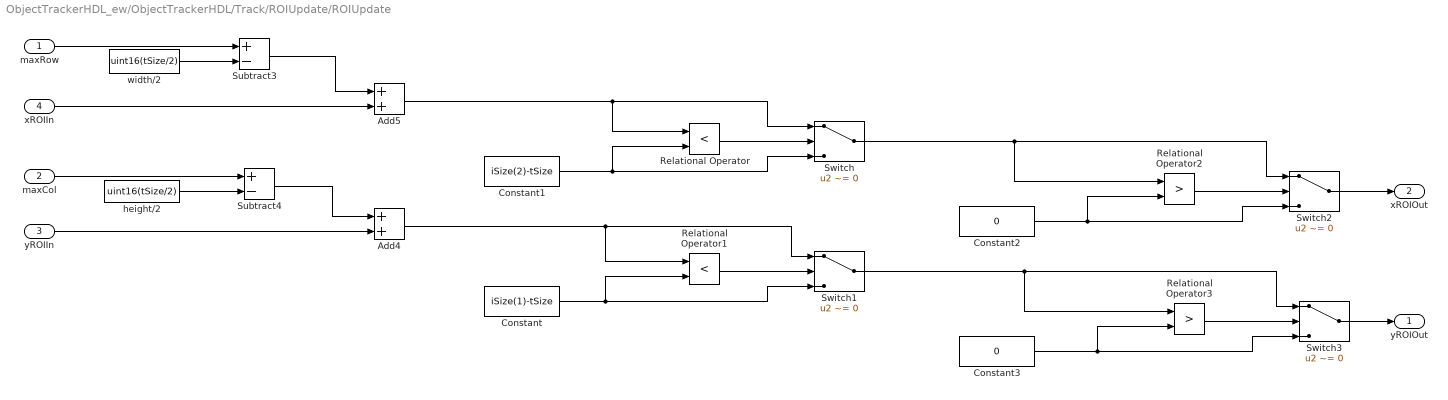
== system ObjectTrackerHDL_ew/ObjectTrackerHDL/Track/ROIUpdate/ROIUpdate ==
  maxRow : Inport
  maxCol : Inport  Port=2
  yROIIn : Inport  Port=3
  xROIIn : Inport  Port=4
  Add4 : Sum  OutDataTypeStr=fixdt(1,17,0)
  Add5 : Sum  OutDataTypeStr=fixdt(1,17,0)
  Constant : Constant  Value=iSize(1)-tSize  OutDataTypeStr=fixdt(1,17,0)  SampleTime=-1
  Constant1 : Constant  Value=iSize(2)-tSize  OutDataTypeStr=fixdt(1,17,0)  SampleTime=-1
  Constant2 : Constant  Value=0  OutDataTypeStr=fixdt(1,17,0)  SampleTime=-1
  Constant3 : Constant  Value=0  OutDataTypeStr=fixdt(1,17,0)  SampleTime=-1
  Relational Operator : RelationalOperator  Operator=<  OutDataTypeStr=boolean  RndMeth=Simplest  InputSameDT=off
  Relational Operator1 : RelationalOperator  Operator=<  OutDataTypeStr=boolean  RndMeth=Simplest  InputSameDT=off
  Relational Operator2 : RelationalOperator  Operator=>  OutDataTypeStr=boolean  RndMeth=Simplest  InputSameDT=off
  Relational Operator3 : RelationalOperator  Operator=>  OutDataTypeStr=boolean  RndMeth=Simplest  InputSameDT=off
  Subtract3 : Sum  Inputs=+-  OutDataTypeStr=fixdt(1,17,0)
  Subtract4 : Sum  Inputs=+-  OutDataTypeStr=fixdt(1,17,0)
  Switch{,1..3} (4 alike) : Switch  Criteria=u2 ~= 0  SaturateOnIntegerOverflow=off  InputSameDT=off
  height/2 : Constant  Value=uint16(tSize/2)  SampleTime=-1
  width/2 : Constant  Value=uint16(tSize/2)  SampleTime=-1
  yROIOut : Outport
  xROIOut : Outport  Port=2
  wires:
  width/2/1 -> Subtract3/2
  Subtract3/1 -> Add5/1
  height/2/1 -> Subtract4/2
  maxRow/1 -> Subtract3/1
  Subtract4/1 -> Add4/1
  maxCol/1 -> Subtract4/1
  yROIIn/1 -> Add4/2
  xROIIn/1 -> Add5/2
  Constant1/1 -> Relational Operator/2, Switch/3
  Switch/1 -> Switch2/1, Relational Operator2/1
  Add5/1 -> Switch/1, Relational Operator/1
  Relational Operator/1 -> Switch/2
  Add4/1 -> Switch1/1, Relational Operator1/1
  Constant/1 -> Switch1/3, Relational Operator1/2
  Relational Operator1/1 -> Switch1/2
  Relational Operator2/1 -> Switch2/2
  Constant2/1 -> Relational Operator2/2, Switch2/3
  Switch2/1 -> xROIOut/1
  Switch1/1 -> Switch3/1, Relational Operator3/1
  Relational Operator3/1 -> Switch3/2
  Switch3/1 -> yROIOut/1
  Constant3/1 -> Relational Operator3/2, Switch3/3

== system ObjectTrackerHDL_ew/ObjectTrackerHDL/Track/2-DCorrelation/2-DIFFT/CornerTurnMemory ==
  dataIn : Inport
  validIn : Inport  Port=2
  BankBit : Subsystem
  Bit Slice3 : hdlsllib/Logic and Bit Operations/Bit Slice  lidx=(log2(numCols)+log2(numRows))-1  ridx=0
  CounterDelay : MATLAB Function  TreatAsAtomicUnit=on  mask{DELAY=tSize*tSize, templateSize=tSize, blanking=tSize+44}
      mask prompts: templateSize "Template Size"
  Delay : Delay  DelayLength=1
  Delay1 : Delay  DelayLength=1
  Logical Operator3 : Logic  IconShape=distinctive  AllPortsSameDT=off  OutDataTypeStr=boolean
  Logical Operator4 : Logic  IconShape=distinctive  AllPortsSameDT=off  OutDataTypeStr=boolean
  Logical Operator5 : Logic  Operator=NOT  IconShape=distinctive  AllPortsSameDT=off  OutDataTypeStr=boolean
  LowerRAM : Subsystem
  ReadAddrCntr : hdlsllib/Sources/HDL Counter  CountType=Count limited  CountInit=0  CountStep=1  CountMax=(2 * numCols * numRows) -1  CountFromType=Initial value  CountFrom=0  CountResetPort=off  CountLoadPort=off  CountEnbPort=on  CountDirPort=off  CountHitOutputPort=off  CountDataType=Unsigned  CountWordLen=log2(numCols) + log2(numRows) + 1  CountFracLen=0  CountSampTime=-1
  SwapAddr : Subsystem
  Switch1 : Switch  Criteria=u2 ~= 0  SaturateOnIntegerOverflow=off  InputSameDT=off
  UpperRAM : Subsystem
  WriteAddrCntr : hdlsllib/Sources/HDL Counter  CountType=Count limited  CountInit=0  CountStep=1  CountMax=(2 * numCols * numRows)-1  CountFromType=Initial value  CountFrom=0  CountResetPort=off  CountLoadPort=off  CountEnbPort=on  CountDirPort=off  CountHitOutputPort=off  CountDataType=Unsigned  CountWordLen=log2(numCols) + log2(numRows) + 1  CountFracLen=0  CountSampTime=-1
  dataOut : Outport
  validOut : Outport  Port=2
  wires:
  CounterDelay/1(vld_out) -> Delay1/1, ReadAddrCntr/1
  Logical Operator4/1 -> UpperRAM/3(wr_en)  "enbWrUp"
  SwapAddr/2(addrRd) -> UpperRAM/4(rd_addr), LowerRAM/4(rd_addr)  "addrRd"
  validIn/1 -> WriteAddrCntr/1, CounterDelay/1(vld_in), Logical Operator4/2, Logical Operator3/1
  Bit Slice3/1 -> UpperRAM/2(wr_addr), LowerRAM/2(wr_addr)  "addrWr"
  WriteAddrCntr/1 -> Bit Slice3/1, BankBit/1(addrIn)  "writeAddr"
  Logical Operator3/1 -> LowerRAM/3(wr_en)  "enbWrLo"
  ReadAddrCntr/1 -> SwapAddr/1(addrIn)  "readAddr"
  LowerRAM/1(dout) -> Switch1/1
  SwapAddr/1(bankRd) -> Delay/1
  UpperRAM/1(dout) -> Switch1/3
  dataIn/1 -> UpperRAM/1(din), LowerRAM/1(din)
  Delay/1 -> Switch1/2
  Logical Operator5/1 -> Logical Operator4/1
  BankBit/1(bankWr) -> Logical Operator5/1, Logical Operator3/2
  Switch1/1 -> dataOut/1  "dataOut"
  Delay1/1 -> validOut/1  "validOut"

== system ObjectTrackerHDL_ew/ObjectTrackerHDL/Track/2-DCorrelation/2-DIFFT/pixelBusGenerator ==
  validIn : Inport
  Horizontal : hdlsllib/Sources/HDL Counter  CountType=Count limited  CountInit=0  CountStep=1  CountMax=hEnd  CountFromType=Initial value  CountFrom=0  CountResetPort=off  CountLoadPort=off  CountEnbPort=on  CountDirPort=off  CountHitOutputPort=off  CountDataType=Unsigned  CountWordLen=ceil(log2(hEnd))  CountFracLen=0  CountSampTime=1
  Logical Operator{3..6} (4 alike) : Logic  AllPortsSameDT=off  OutDataTypeStr=boolean
  Pixel Control Bus Creator : visionhdlutilities/Pixel Control Bus Creator
  Vertical : hdlsllib/Sources/HDL Counter  CountType=Count limited  CountInit=0  CountStep=1  CountMax=vEnd  CountFromType=Initial value  CountFrom=0  CountResetPort=off  CountLoadPort=off  CountEnbPort=on  CountDirPort=off  CountHitOutputPort=off  CountDataType=Unsigned  CountWordLen=ceil(log2(vEnd))  CountFracLen=0  CountSampTime=1
  hEnd : simulink/Logic and Bit Operations/Compare To Constant  relop===  const=hEnd  OutDataTypeStr=boolean
  hStart : simulink/Logic and Bit Operations/Compare To Constant  relop===  const=0  OutDataTypeStr=boolean
  vEnd : simulink/Logic and Bit Operations/Compare To Constant  relop===  const=vEnd  OutDataTypeStr=boolean
  vStart : simulink/Logic and Bit Operations/Compare To Constant  relop===  const=0  OutDataTypeStr=boolean
  busOut : Outport  VectorParamsAs1DForOutWhenUnconnected=off
  frameDone : Outport  Port=2  VectorParamsAs1DForOutWhenUnconnected=off
  wires:
  validIn/1 -> Pixel Control Bus Creator/5, Vertical/1, Logical Operator4/1, Logical Operator5/1, Logical Operator6/1, Logical Operator3/1, Horizontal/1
  Horizontal/1 -> hEnd/1, hStart/1
  hEnd/1 -> Logical Operator4/2
  Vertical/1 -> vStart/1, vEnd/1
  vStart/1 -> Logical Operator5/2
  vEnd/1 -> Logical Operator6/2
  Logical Operator5/1 -> Pixel Control Bus Creator/3
  Logical Operator3/1 -> Pixel Control Bus Creator/1
  Logical Operator4/1 -> Pixel Control Bus Creator/2
  hStart/1 -> Logical Operator3/2
  Logical Operator6/1 -> frameDone/1, Pixel Control Bus Creator/4
  Pixel Control Bus Creator/1 -> busOut/1

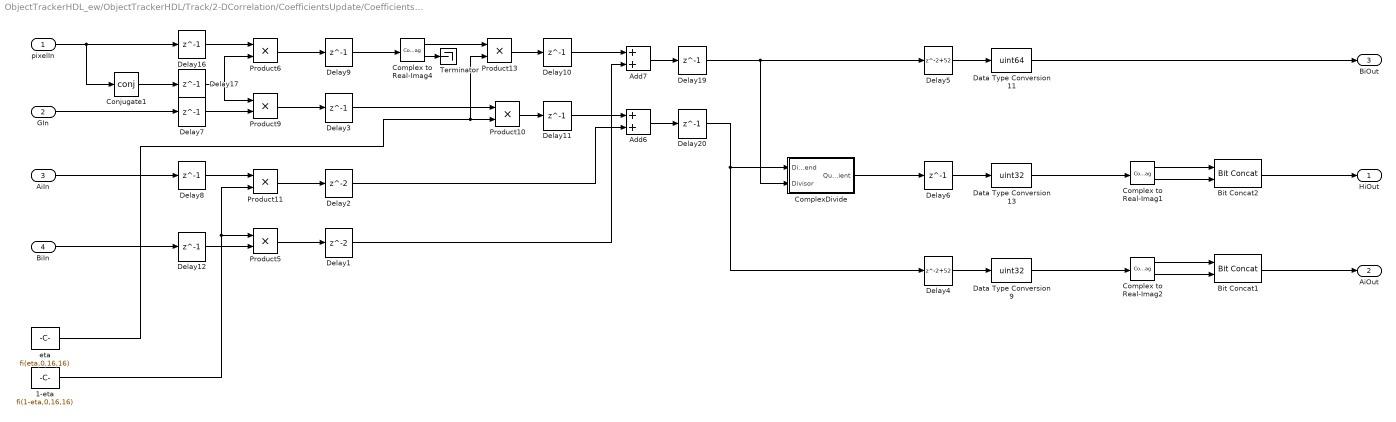
== system ObjectTrackerHDL_ew/ObjectTrackerHDL/Track/2-DCorrelation/CoefficientsUpdate/CoefficientsUpdate ==
  pixelIn : Inport
  GIn : Inport  Port=2
  AiIn : Inport  Port=3
  BiIn : Inport  Port=4
  1-eta : Constant  Value=fi(1-eta,0,16,16)  OutDataTypeStr=fixdt(0,16,16)  SampleTime=-1
  Add6 : Sum  OutDataTypeStr=fixdt(1,28,8)
  Add7 : Sum  OutDataTypeStr=fixdt(1,36,8)
  Bit Concat1 : hdlsllib/Logic and Bit Operations/Bit Concat  numInputs=2
  Bit Concat2 : hdlsllib/Logic and Bit Operations/Bit Concat  numInputs=2
  Complex to Real-Imag1 : ComplexToRealImag
  Complex to Real-Imag2 : ComplexToRealImag
  Complex to Real-Imag4 : ComplexToRealImag
  ComplexDivide : Subsystem
  Conjugate1 : Math  Operator=conj  SignedPower=on  RndMeth=Zero
  Data Type Conversion11 : DataTypeConversion  OutDataTypeStr=uint64  ConvertRealWorld=Stored Integer (SI)  SaturateOnIntegerOverflow=off  RndMeth=Floor
  Data Type Conversion13 : DataTypeConversion  OutDataTypeStr=uint32  ConvertRealWorld=Stored Integer (SI)  SaturateOnIntegerOverflow=off  RndMeth=Floor
  Data Type Conversion9 : DataTypeConversion  OutDataTypeStr=uint32  ConvertRealWorld=Stored Integer (SI)  SaturateOnIntegerOverflow=off  RndMeth=Floor
  Delay1 : Delay  InitialCondition=0
  Delay{3,6..12,16..17,19..20} (12 alike) : Delay  DelayLength=1  InitialCondition=0
  Delay2 : Delay  InitialCondition=0
  Delay4 : Delay  DelayLength=2+52  InitialCondition=0
  Delay5 : Delay  DelayLength=2+52  InitialCondition=0
  Product10 : Product  OutDataTypeStr=fixdt(1,24,12)
  Product11 : Product  OutDataTypeStr=fixdt(1,28,8)
  Product13 : Product  OutDataTypeStr=fixdt(1,32,12)
  Product5 : Product  OutDataTypeStr=fixdt(1,36,8)
  Product6 : Product  OutDataTypeStr=fixdt(1,32,8)
  Product9 : Product  OutDataTypeStr=fixdt(1,24,8)
  Terminator : Terminator
  eta : Constant  Value=fi(eta,0,16,16)  SampleTime=-1
  HiOut : Outport
  AiOut : Outport  Port=2
  BiOut : Outport  Port=3
  wires:
  Delay19/1 -> ComplexDivide/2(Divisor), Delay5/1
  Delay6/1 -> Data Type Conversion13/1
  Delay4/1 -> Data Type Conversion9/1
  Delay2/1 -> Add6/2
  Complex to Real-Imag4/2 -> Terminator/1
  Delay3/1 -> Product10/1
  Delay20/1 -> Delay4/1, ComplexDivide/1(Dividend)
  Data Type Conversion9/1 -> Complex to Real-Imag2/1
  Complex to Real-Imag2/1 -> Bit Concat1/1
  BiIn/1 -> Delay12/1
  Delay11/1 -> Add6/1
  AiIn/1 -> Delay8/1
  Delay5/1 -> Data Type Conversion11/1
  eta/1 -> Product13/2, Product10/2
  Delay9/1 -> Complex to Real-Imag4/1
  Data Type Conversion13/1 -> Complex to Real-Imag1/1
  Conjugate1/1 -> Delay17/1
  Product11/1 -> Delay2/1
  Product13/1 -> Delay10/1
  1-eta/1 -> Product5/1, Product11/2
  Add7/1 -> Delay19/1
  Complex to Real-Imag4/1 -> Product13/1
  Product9/1 -> Delay3/1
  Add6/1 -> Delay20/1
  pixelIn/1 -> Delay16/1, Conjugate1/1
  Product10/1 -> Delay11/1
  Delay17/1 -> Product9/1, Product6/2
  Complex to Real-Imag1/1 -> Bit Concat2/1
  Delay1/1 -> Add7/2
  Delay10/1 -> Add7/1
  Delay16/1 -> Product6/1
  Product5/1 -> Delay1/1
  Complex to Real-Imag2/2 -> Bit Concat1/2
  GIn/1 -> Delay7/1
  Complex to Real-Imag1/2 -> Bit Concat2/2
  Product6/1 -> Delay9/1
  Bit Concat1/1 -> AiOut/1
  Data Type Conversion11/1 -> BiOut/1
  Bit Concat2/1 -> HiOut/1
  ComplexDivide/1(Quotient) -> Delay6/1
  Delay7/1 -> Product9/2
  Delay8/1 -> Product11/1
  Delay12/1 -> Product5/2

== system ObjectTrackerHDL_ew/ObjectTrackerHDL/Track/2-DCorrelation/Curr2-DFFT/CornerTurnMemory ==
  dataIn : Inport
  validIn : Inport  Port=2
  BankBit : Subsystem
  Bit Slice : hdlsllib/Logic and Bit Operations/Bit Slice  lidx=(log2(numCols)+log2(numRows))-1  ridx=0
  CounterDelay : MATLAB Function  TreatAsAtomicUnit=on  mask{DELAY=tSize*tSize, templateSize=tSize, blanking=tSize+44}
      mask prompts: templateSize "Template Size"
  Delay : Delay  DelayLength=1
  Delay1 : Delay  DelayLength=1
  Logical Operator : Logic  IconShape=distinctive  AllPortsSameDT=off  OutDataTypeStr=boolean
  Logical Operator1 : Logic  IconShape=distinctive  AllPortsSameDT=off  OutDataTypeStr=boolean
  Logical Operator2 : Logic  Operator=NOT  IconShape=distinctive  AllPortsSameDT=off  OutDataTypeStr=boolean
  LowerRAM : Subsystem
  ReadAddrCntr : hdlsllib/Sources/HDL Counter  CountType=Count limited  CountInit=0  CountStep=1  CountMax=(2 * numCols * numRows) -1  CountFromType=Initial value  CountFrom=0  CountResetPort=off  CountLoadPort=off  CountEnbPort=on  CountDirPort=off  CountHitOutputPort=off  CountDataType=Unsigned  CountWordLen=log2(numCols) + log2(numRows) + 1  CountFracLen=0  CountSampTime=-1
  SwapAddr : Subsystem
  Switch : Switch  Criteria=u2 ~= 0  SaturateOnIntegerOverflow=off  InputSameDT=off
  UpperRAM : Subsystem
  WriteAddrCntr : hdlsllib/Sources/HDL Counter  CountType=Count limited  CountInit=0  CountStep=1  CountMax=(2 * numCols * numRows)-1  CountFromType=Initial value  CountFrom=0  CountResetPort=off  CountLoadPort=off  CountEnbPort=on  CountDirPort=off  CountHitOutputPort=off  CountDataType=Unsigned  CountWordLen=log2(numCols) + log2(numRows) + 1  CountFracLen=0  CountSampTime=-1
  dataOut : Outport
  validOut : Outport  Port=2
  wires:
  BankBit/1(bankWr) -> Logical Operator2/1, Logical Operator/2
  dataIn/1 -> LowerRAM/1(din), UpperRAM/1(din)
  ReadAddrCntr/1 -> SwapAddr/1(addrIn)  "readAddr"
  Bit Slice/1 -> UpperRAM/2(wr_addr), LowerRAM/2(wr_addr)  "addrWr"
  Logical Operator/1 -> LowerRAM/3(wr_en)  "enbWrLo"
  Logical Operator2/1 -> Logical Operator1/1
  WriteAddrCntr/1 -> Bit Slice/1, BankBit/1(addrIn)  "writeAddr"
  Switch/1 -> dataOut/1  "dataOut"
  Delay1/1 -> validOut/1  "validOut"
  SwapAddr/1(bankRd) -> Delay/1
  Logical Operator1/1 -> UpperRAM/3(wr_en)  "enbWrUp"
  LowerRAM/1(dout) -> Switch/1
  UpperRAM/1(dout) -> Switch/3
  SwapAddr/2(addrRd) -> UpperRAM/4(rd_addr), LowerRAM/4(rd_addr)  "addrRd"
  CounterDelay/1(vld_out) -> Delay1/1, ReadAddrCntr/1
  validIn/1 -> WriteAddrCntr/1, Logical Operator/1, CounterDelay/1(vld_in), Logical Operator1/2
  Delay/1 -> Switch/2

== system ObjectTrackerHDL_ew/ObjectTrackerHDL/Track/2-DCorrelation/Curr2-DFFT/pixelBusGenerator ==
  validIn : Inport
  Horizontal : hdlsllib/Sources/HDL Counter  CountType=Count limited  CountInit=0  CountStep=1  CountMax=hEnd  CountFromType=Initial value  CountFrom=0  CountResetPort=off  CountLoadPort=off  CountEnbPort=on  CountDirPort=off  CountHitOutputPort=off  CountDataType=Unsigned  CountWordLen=ceil(log2(hEnd))  CountFracLen=0  CountSampTime=1
  Logical Operator{3..6} (4 alike) : Logic  AllPortsSameDT=off  OutDataTypeStr=boolean
  Pixel Control Bus Creator : visionhdlutilities/Pixel Control Bus Creator
  Vertical : hdlsllib/Sources/HDL Counter  CountType=Count limited  CountInit=0  CountStep=1  CountMax=vEnd  CountFromType=Initial value  CountFrom=0  CountResetPort=off  CountLoadPort=off  CountEnbPort=on  CountDirPort=off  CountHitOutputPort=off  CountDataType=Unsigned  CountWordLen=ceil(log2(vEnd))  CountFracLen=0  CountSampTime=1
  hEnd : simulink/Logic and Bit Operations/Compare To Constant  relop===  const=hEnd  OutDataTypeStr=boolean
  hStart : simulink/Logic and Bit Operations/Compare To Constant  relop===  const=0  OutDataTypeStr=boolean
  vEnd : simulink/Logic and Bit Operations/Compare To Constant  relop===  const=vEnd  OutDataTypeStr=boolean
  vStart : simulink/Logic and Bit Operations/Compare To Constant  relop===  const=0  OutDataTypeStr=boolean
  busOut : Outport  VectorParamsAs1DForOutWhenUnconnected=off
  frameDone : Outport  Port=2  VectorParamsAs1DForOutWhenUnconnected=off
  wires:
  validIn/1 -> Pixel Control Bus Creator/5, Vertical/1, Logical Operator4/1, Logical Operator5/1, Logical Operator6/1, Logical Operator3/1, Horizontal/1
  Horizontal/1 -> hEnd/1, hStart/1
  hEnd/1 -> Logical Operator4/2
  Vertical/1 -> vStart/1, vEnd/1
  vStart/1 -> Logical Operator5/2
  vEnd/1 -> Logical Operator6/2
  Logical Operator5/1 -> Pixel Control Bus Creator/3
  Logical Operator3/1 -> Pixel Control Bus Creator/1
  Logical Operator4/1 -> Pixel Control Bus Creator/2
  hStart/1 -> Logical Operator3/2
  Logical Operator6/1 -> frameDone/1, Pixel Control Bus Creator/4
  Pixel Control Bus Creator/1 -> busOut/1

== system ObjectTrackerHDL_ew/ObjectTrackerHDL/Track/2-DCorrelation/Prev2-DFFT/CornerTurnMemory ==
  dataIn : Inport
  validIn : Inport  Port=2
  BankBit : Subsystem
  Bit Slice : hdlsllib/Logic and Bit Operations/Bit Slice  lidx=(log2(numCols)+log2(numRows))-1  ridx=0
  CounterDelay : MATLAB Function  TreatAsAtomicUnit=on  mask{DELAY=tSize*tSize, templateSize=tSize, blanking=tSize+44}
      mask prompts: templateSize "Template Size"
  Delay : Delay  DelayLength=1
  Delay1 : Delay  DelayLength=1
  Logical Operator : Logic  IconShape=distinctive  AllPortsSameDT=off  OutDataTypeStr=boolean
  Logical Operator1 : Logic  IconShape=distinctive  AllPortsSameDT=off  OutDataTypeStr=boolean
  Logical Operator2 : Logic  Operator=NOT  IconShape=distinctive  AllPortsSameDT=off  OutDataTypeStr=boolean
  LowerRAM : Subsystem
  ReadAddrCntr : hdlsllib/Sources/HDL Counter  CountType=Count limited  CountInit=0  CountStep=1  CountMax=(2 * numCols * numRows) -1  CountFromType=Initial value  CountFrom=0  CountResetPort=off  CountLoadPort=off  CountEnbPort=on  CountDirPort=off  CountHitOutputPort=off  CountDataType=Unsigned  CountWordLen=log2(numCols) + log2(numRows) + 1  CountFracLen=0  CountSampTime=-1
  SwapAddr : Subsystem
  Switch : Switch  Criteria=u2 ~= 0  SaturateOnIntegerOverflow=off  InputSameDT=off
  UpperRAM : Subsystem
  WriteAddrCntr : hdlsllib/Sources/HDL Counter  CountType=Count limited  CountInit=0  CountStep=1  CountMax=(2 * numCols * numRows)-1  CountFromType=Initial value  CountFrom=0  CountResetPort=off  CountLoadPort=off  CountEnbPort=on  CountDirPort=off  CountHitOutputPort=off  CountDataType=Unsigned  CountWordLen=log2(numCols) + log2(numRows) + 1  CountFracLen=0  CountSampTime=-1
  dataOut : Outport
  validOut : Outport  Port=2
  wires:
  BankBit/1(bankWr) -> Logical Operator2/1, Logical Operator/2
  ReadAddrCntr/1 -> SwapAddr/1(addrIn)  "readAddr"
  Bit Slice/1 -> UpperRAM/2(wr_addr), LowerRAM/2(wr_addr)  "addrWr"
  Logical Operator/1 -> LowerRAM/3(wr_en)  "enbWrLo"
  Logical Operator2/1 -> Logical Operator1/1
  WriteAddrCntr/1 -> Bit Slice/1, BankBit/1(addrIn)  "writeAddr"
  Switch/1 -> dataOut/1  "dataOut"
  Delay1/1 -> validOut/1  "validOut"
  SwapAddr/1(bankRd) -> Delay/1
  Logical Operator1/1 -> UpperRAM/3(wr_en)  "enbWrUp"
  LowerRAM/1(dout) -> Switch/1
  UpperRAM/1(dout) -> Switch/3
  SwapAddr/2(addrRd) -> UpperRAM/4(rd_addr), LowerRAM/4(rd_addr)  "addrRd"
  CounterDelay/1(vld_out) -> Delay1/1, ReadAddrCntr/1
  validIn/1 -> WriteAddrCntr/1, Logical Operator/1, CounterDelay/1(vld_in), Logical Operator1/2
  Delay/1 -> Switch/2
  dataIn/1 -> LowerRAM/1(din), UpperRAM/1(din)
